simulink model "prob4"  (R2020b)
settings: Solver=FixedStepDiscrete  StartTime=0.0  StopTime=10.0  MaxStep=0.001  RelTol=1e-3
model workspace: external: MATLAB File C:\Users\deves\MATLAB\Projects\problem4\data.m (data not in the file)
undefined symbols (not defined in the file): a1, a2, b0, b1
settings Model: Creator=deves  LastModifiedBy=deves

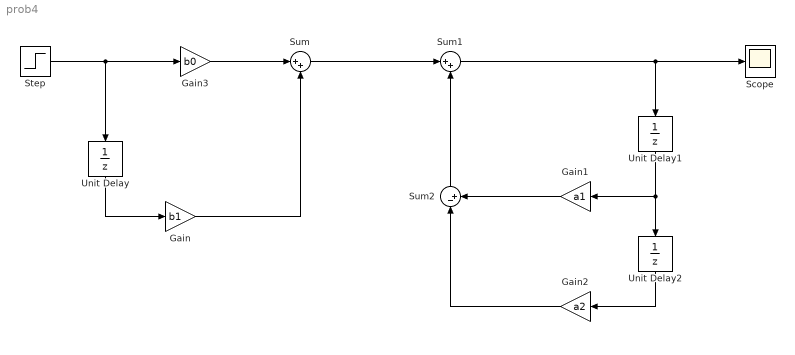
== system prob4 ==
  Gain : Gain  Gain=b1
  Gain1 : Gain  Gain=a1
  Gain2 : Gain  Gain=a2
  Gain3 : Gain  Gain=b0
  Scope : Scope
  Step : Step  SampleTime=0
  Sum : Sum  Inputs=|++
  Sum1 : Sum  Inputs=|++
  Sum2 : Sum  Inputs=|-+
  Unit Delay : UnitDelay  SampleTime=-1  HasFrameUpgradeWarning=on
  Unit Delay1 : UnitDelay  SampleTime=-1  HasFrameUpgradeWarning=on
  Unit Delay2 : UnitDelay  SampleTime=-1  HasFrameUpgradeWarning=on
  wires:
  Step/1 -> Gain3/1, Unit Delay/1
  Unit Delay/1 -> Gain/1
  Gain/1 -> Sum/2
  Sum/1 -> Sum1/1
  Unit Delay1/1 -> Gain1/1, Unit Delay2/1
  Unit Delay2/1 -> Gain2/1
  Gain1/1 -> Sum2/2
  Gain2/1 -> Sum2/1
  Sum2/1 -> Sum1/2
  Sum1/1 -> Unit Delay1/1, Scope/1
  Gain3/1 -> Sum/1
